simulink model "Q3_Block"  (R2018a)
settings: Solver=VariableStepAuto  StartTime=0.0  StopTime=400  RelTol=1e-3
settings Model: Creator=lab User  LastModifiedBy=lab User

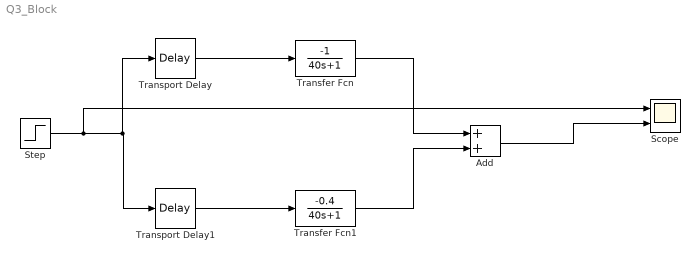
== system Q3_Block ==
  Add : Sum
  Scope : Scope  NumInputPorts=2
  Step : Step  SampleTime=0
  Transfer Fcn : TransferFcn  Numerator=[-1]  Denominator=[40 1]
  Transfer Fcn1 : TransferFcn  Numerator=[-0.4]  Denominator=[40 1]
  Transport Delay : TransportDelay  DelayTime=30
  Transport Delay1 : TransportDelay  DelayTime=75
  wires:
  Transport Delay/1 -> Transfer Fcn/1
  Transport Delay1/1 -> Transfer Fcn1/1
  Transfer Fcn/1 -> Add/1
  Transfer Fcn1/1 -> Add/2
  Step/1 -> Scope/1, Transport Delay/1, Transport Delay1/1
  Add/1 -> Scope/2
